simulink model "modelo_planta_CODESYS"  (R2025b)
settings: Solver=FixedStepAuto  StartTime=0.0  StopTime=inf  FixedStep=Ts2  MaxStep=1e-3  RelTol=1e-3
undefined symbols (not defined in the file): ah_max, at_max, bcx, bcy, bh_eq, bhb, bhEb, bhwu, bt, bt_eq, btb, btw, g, Hc, ih, it, Jh_eq, Jt_eq, Kcy, khwu, Ki_h, Ki_t, Kp_h, Kp_t, Kpos_h, Kpos_t, Ktw, lambda, Lh, Lh0, lh_0, Lt, magnitude, Mc_max, Ms, Mt, rhd, rtd, tau_hm, tau_tm, Thb_Max, ThEb_Max, Thm_0, Thm_Max, titahm_0, titatm_0, Ts0, Ts1, Ts2, Ttb_Max, Ttm_0, Ttm_Max, vh_0, vlx_0, vly_0, vt_0, vt_max, Wc, whm_0, whm_rated ... (+11)
libraries: simulink x10, opcualib x7, sl3dlib x1, simulink_extras x1, dspnetwork x1
(part 2 of 2)

== system modelo_planta_CODESYS/Subsistema Izaje/Dinámica carga izaje/Lógica Masa y Altura ==
  McX : Inport
  TLK : Inport  Port=2
  Constant : Constant  Value=Ms
  Constant1 : Constant  Value=0
  Constant2 : Constant  Value=Hc
  Rate Limiter : RateLimiter  Commented=through  RisingSlewLimit=Mc_max/0.1  FallingSlewLimit=-Mc_max/0.1  SampleTimeMode=inherited  InitialCondition=Ms
  Sum1 : Sum  Inputs=|++
  Switch : Switch  Criteria=u2 > Threshold  SaturateOnIntegerOverflow=off  InputSameDT=off
  Switch1 : Switch  Criteria=u2 > Threshold  SaturateOnIntegerOverflow=off  InputSameDT=off
  ml : Outport
  hc : Outport  Port=2
  wires:
  Sum1/1 -> Switch/1
  Constant2/1 -> Switch1/1
  TLK/1 -> Switch1/2, Switch/2
  Constant/1 -> Switch/3, Sum1/2
  Constant1/1 -> Switch1/3
  McX/1 -> Sum1/1
  Switch/1 -> Rate Limiter/1
  Rate Limiter/1 -> ml/1
  Switch1/1 -> hc/1

== system modelo_planta_CODESYS/Subsistema Izaje/Dinámica carga izaje/Lógica contacto ==
  delta_y : Inport
  vlx : Inport  Port=2
  vly : Inport  Port=3
  Constant3 : Constant  Value=0
  Constant4 : Constant  Value=0
  Gain3 : Gain  Gain=Kcy
  Gain4 : Gain  Gain=bcy
  Gain5 : Gain  Gain=-bcx
  Saturation : Saturate  UpperLimit=60e5  LowerLimit=0
  Sum5 : Sum  Inputs=-+|
  Switch2 : Switch  SaturateOnIntegerOverflow=off  InputSameDT=off
  Switch3 : Switch  SaturateOnIntegerOverflow=off  InputSameDT=off
  Fcy : Outport
  Fcx : Outport  Port=2
  wires:
  Sum5/1 -> Switch2/1
  vlx/1 -> Gain5/1
  Gain4/1 -> Sum5/1
  vly/1 -> Gain4/1
  Constant4/1 -> Switch3/3
  Gain5/1 -> Switch3/1
  Gain3/1 -> Sum5/2
  delta_y/1 -> Switch3/2, Gain3/1, Switch2/2
  Constant3/1 -> Switch2/3
  Switch2/1 -> Saturation/1  "Fcy"
  Switch3/1 -> Fcx/1  "Fcx"
  Saturation/1 -> Fcy/1

== matlab function modelo_planta_CODESYS/Controlador Carro v2/MATLAB Function ==
  data: tita_l input; v_sway output; yh_enc input; m_est input; Yt0 parameter; g parameter; lambda parameter; Ms parameter; Mc_max parameter; antisway input
function v_sway = Control_Balanceo(tita_l, yh_enc, m_est, Yt0, g, lambda, Ms, Mc_max, antisway)
    
    % 1. Compensación de inercia (ganancia_masa)
    L_vacio = 1.0;
    L_lleno = 0.6;
    
    factor = (m_est - Ms) / Mc_max;
    factor = max(0, min(1, factor)); % Saturación entre 0 y 1
    
    g_masa = L_vacio + (L_lleno - L_vacio) * factor;

    % 2. Cinemática del péndulo
    % Longitud del cable (l)
    l_pendulo = Yt0 - yh_enc;
    
    % Ganancia cinemática
    K_cinematico = 2 * lambda * g_masa * sqrt(abs(g * l_pendulo));

    % 3. Multiplicación por el ángulo y activación del bloque
    v_sway = tita_l * K_cinematico * antisway;
end

== matlab function modelo_planta_CODESYS/Controlador Carro v2/MATLAB Function1 ==
  data: x_ref_s output; xt_ref input; vt_max parameter; at_max parameter; v_ref_s output; Ts2 parameter; xt_0 parameter; vt_0 parameter
function [x_ref_s, v_ref_s] = Curva_S_t(xt_ref, vt_max, at_max, Ts2, xt_0, vt_0)
    % Memorias (Equivalente a los bloques Z^-1)
    persistent x_ref_s_prev v_ref_s_prev
    
    % Inicialización en el primer ciclo
    if isempty(x_ref_s_prev)
        x_ref_s_prev = xt_0;
        v_ref_s_prev = vt_0;
    end
    
    % 1. Sumador de entrada (Error de posición)
    error_pos = xt_ref - x_ref_s_prev;
    
    % 2. Frenado Óptimo
    d_tol = 0.1;
    if abs(error_pos) > d_tol
        vh_brakes = sqrt(2 * at_max * abs(error_pos));
        vt_cmd = vh_brakes * sign(error_pos);
    else
        vh_limit_tol = sqrt(2 * at_max * d_tol);
        gain_linear = vh_limit_tol / d_tol;      
        vt_cmd = gain_linear * error_pos;
    end
    
    % 3. Saturación (Limitar la velocidad máxima)
    vt_cmd_sat = max(-vt_max, min(vt_max, vt_cmd));
    
    % 4. Rate Limiter
    delta_v = vt_cmd_sat - v_ref_s_prev;
    limite_delta = at_max * Ts2; % Cuánto puede cambiar la velocidad en 1 ciclo
    
    delta_v_limitado = max(-limite_delta, min(limite_delta, delta_v));
    v_ref_s = v_ref_s_prev + delta_v_limitado;
    
    % 5. Integrador Discreto (Tustin)
    x_ref_s = x_ref_s_prev + (Ts2 / 2) * (v_ref_s + v_ref_s_prev);
    
    % 6. Actualizar memorias para el siguiente ciclo
    v_ref_s_prev = v_ref_s;
    x_ref_s_prev = x_ref_s;
end

== matlab function modelo_planta_CODESYS/Controlador Carro v2/MATLAB Function2 ==
  data: vx_cmd input; vt_ref output; modo_manual input; x_ref_s input; v_ref_s input; xtd_enc input; v_sway input; vt_0 parameter; Ts2 parameter; at_max parameter; vt_max parameter; Kpos_t parameter
function vt_ref = Lazo_Externo_t(vx_cmd, modo_manual, x_ref_s, v_ref_s, xtd_enc, v_sway, vt_0, Ts2, at_max, vt_max, Kpos_t)
    % Memoria
    persistent vt_ref_prev
    
    if isempty(vt_ref_prev)
        vt_ref_prev = vt_0;
    end

    % 1. Control de posición automático
    e_x = x_ref_s - xtd_enc;
    vel_auto = (e_x * Kpos_t) + (v_ref_s * 0.5);

    % 2. Selector de Modo
    % Si modo_manual es true (1), pasa la señal manual, si no, la automática
    if modo_manual > 0 
        vel_base = vx_cmd;
    else
        vel_base = vel_auto;
    end

    % 3. Suma del Anti-Sway
    vt_cmd = vel_base + v_sway;

    % 4. Límite de Velocidad
    vt_cmd_sat = max(-vt_max, min(vt_max, vt_cmd));

    % 5. Límite de Aceleración
    delta_v = vt_cmd_sat - vt_ref_prev;
    limite_delta = at_max * Ts2;
    
    delta_v_limitado = max(-limite_delta, min(limite_delta, delta_v));
    vt_ref = vt_ref_prev + delta_v_limitado;

    % 6. Actualizar memoria
    vt_ref_prev = vt_ref;
end

== matlab function modelo_planta_CODESYS/Controlador Carro v2/MATLAB Function3 ==
  data: xtd_enc input; vt_obs output; Ttm_ref input; wtm_0 parameter; titatm_0 parameter; Lt parameter; bt_eq parameter; Jt_eq parameter; rtd parameter; it parameter; Ts2 parameter
function vt_obs = Observador_Estado_t(xtd_enc, Ttm_ref, wtm_0, titatm_0, Lt, bt_eq, Jt_eq, rtd, it, Ts2)...
    
    % Memorias
    persistent theta_t_obs_prev wt_obs_prev int_e_prev
    
    % Condiciones iniciales
    if isempty(theta_t_obs_prev)
        theta_t_obs_prev = titatm_0;
        wt_obs_prev      = wtm_0;    
        int_e_prev       = 0.0; 
    end
    
    % 1. Convertir posición lineal del carro a angular del motor
    theta_t_enc = xtd_enc * (it / rtd);
    
    % 2. Error de estimación (Posición real vs observada)
    e_theta_t = theta_t_enc - theta_t_obs_prev;
    
    % 3. Lazo de torque (Física de la planta)
    Torque_net = Ttm_ref - (bt_eq * wt_obs_prev) + (Lt(3) * int_e_prev);
    alpha_phys = Torque_net / Jt_eq; % Aceleración angular
    
    % 4. Derivadas
    dot_wt_obs      = alpha_phys + (Lt(2) * e_theta_t);
    dot_theta_t_obs = wt_obs_prev + (Lt(1) * e_theta_t);

    % 5. Salida del observador
    vt_obs = wt_obs_prev * (rtd / it);
    
    % 6. Integración Discreta
    theta_t_obs = theta_t_obs_prev + (Ts2 * dot_theta_t_obs);
    wt_obs      = wt_obs_prev      + (Ts2 * dot_wt_obs);
    int_e       = int_e_prev       + (Ts2 * e_theta_t);

    % 7. Actualizar memorias para el siguiente ciclo de reloj
    theta_t_obs_prev = theta_t_obs;
    wt_obs_prev      = wt_obs;
    int_e_prev       = int_e;
end

== matlab function modelo_planta_CODESYS/Controlador Carro v2/MATLAB Function4 ==
  data: vt_ref input; Ttm_ref output; vt_obs input; BRK_t input; Ts2 parameter; Ki_t parameter; Kp_t parameter
function Ttm_ref = Lazo_Interno_t(vt_ref, vt_obs, BRK_t, Ts2, Ki_t, Kp_t)
    % Memorias para el integrador
    persistent int_prev e_v_prev
    
    % Inicialización
    if isempty(int_prev)
        int_prev = 0.0;
        e_v_prev = 0.0;
    end
    
    % 1. Cálculo del error de velocidad
    e_v = vt_ref - vt_obs;
    
    % 2. Integrador Discreto (Tustin) con Reset por Freno
    % Si el freno está activo (BRK_t = 0), forzamos la memoria a 0 
    % para evitar la acumulación de error (Anti-Windup).
    if BRK_t > 0
        int_val = int_prev + (Ts2 / 2) * (e_v + e_v_prev);
    else
        int_val = 0.0;
    end
    
    % 3. Controlador PI
    P_out = e_v * Kp_t;
    I_out = int_val * Ki_t;
    
    % Suma final de referencia de torque
    Ttm_ref = P_out + I_out;
    
    % 4. Actualizar memorias
    int_prev = int_val;
    e_v_prev = e_v;
end

== matlab function modelo_planta_CODESYS/Controlador Izaje v2/MATLAB Function1 ==
  data: y_ref_s output; yh_ref input; ah_max parameter; v_ref_s output; Ts2 parameter; yh_0 parameter; vh_0 parameter; vh_lim input
function [y_ref_s, v_ref_s] = Curva_S_h(yh_ref, ah_max, Ts2, yh_0, vh_0, vh_lim)
    % Memorias (Equivalente a los bloques Z^-1)
    persistent x_ref_s_prev v_ref_s_prev
    
    % Inicialización en el primer ciclo
    if isempty(x_ref_s_prev)
        x_ref_s_prev = yh_0;
        v_ref_s_prev = vh_0;
    end
    
    % 1. Sumador de entrada (Error de posición)
    error_pos = yh_ref - x_ref_s_prev;
    
    % 2. Frenado Óptimo
    d_tol = 0.1;
    if abs(error_pos) > d_tol
        vh_brakes = sqrt(2 * ah_max * abs(error_pos));
        vt_cmd = vh_brakes * sign(error_pos);
    else
        vh_limit_tol = sqrt(2 * ah_max * d_tol);
        gain_linear = vh_limit_tol / d_tol;      
        vt_cmd = gain_linear * error_pos;
    end
    
    % 3. Saturación (Limitar la velocidad máxima)
    vt_cmd_sat = max(-vh_lim, min(vh_lim, vt_cmd));
    
    % 4. Rate Limiter
    delta_v = vt_cmd_sat - v_ref_s_prev;
    limite_delta = ah_max * Ts2; % Cuánto puede cambiar la velocidad en 1 ciclo
    
    delta_v_limitado = max(-limite_delta, min(limite_delta, delta_v));
    v_ref_s = v_ref_s_prev + delta_v_limitado;
    
    % 5. Integrador Discreto (Tustin)
    y_ref_s = x_ref_s_prev + (Ts2 / 2) * (v_ref_s + v_ref_s_prev);
    
    % 6. Actualizar memorias para el siguiente ciclo
    v_ref_s_prev = v_ref_s;
    x_ref_s_prev = y_ref_s;
end

== matlab function modelo_planta_CODESYS/Controlador Izaje v2/MATLAB Function2 ==
  data: vy_cmd input; modo_manual input; y_ref_s input; v_ref_s input; vh_lim input; yh_enc input; vh_ref output; Ts2 parameter; ah_max parameter; Kpos_h parameter; vh_0 parameter
function vh_ref = Lazo_Externo_h(vy_cmd, modo_manual, y_ref_s, v_ref_s, vh_lim, yh_enc, Ts2, ah_max, Kpos_h, vh_0)
    % Memoria
    persistent vh_ref_prev
    
    if isempty(vh_ref_prev)
        vh_ref_prev = vh_0;
    end

    % 1. Control de posición automático
    e_y = y_ref_s - yh_enc;
    vel_auto = (e_y * Kpos_h) + (v_ref_s * 0.5);

    % 2. Selector de Modo
    % Si modo_manual es true (1), pasa la señal manual, si no, la automática
    if modo_manual > 0 
        vh_cmd = vy_cmd;
    else
        vh_cmd = vel_auto;
    end

    % 3. Límite de Velocidad
    vh_cmd_sat = max(-vh_lim, min(vh_lim, vh_cmd));

    % 5. Límite de Aceleración
    delta_v = vh_cmd_sat - vh_ref_prev;
    limite_delta = ah_max * Ts2;
    
    delta_v_limitado = max(-limite_delta, min(limite_delta, delta_v));
    vh_ref = vh_ref_prev + delta_v_limitado;

    % 6. Actualizar memoria
    vh_ref_prev = vh_ref;
end

== matlab function modelo_planta_CODESYS/MATLAB Function ==
  data: TLK input; M_carga output; Mc_min parameter
function M_carga = Masa_Aleatoria(TLK, Mc_min)
    persistent masa_actual;
    persistent ultimo_estado_trigger;
    
    % Inicialización
    if isempty(masa_actual)
        masa_actual = Mc_min; % Empezamos con el valor mínimo por defecto
        ultimo_estado_trigger = 0;
    end
    
    % DETECCIÓN DE FLANCO DE SUBIDA (Rising Edge)
    if (TLK == 1 && ultimo_estado_trigger == 0)
        % Generar número aleatorio entre Min y Max
        masa_actual = Mc_min + (55000 - Mc_min) * rand();
        masa_actual = floor(masa_actual); 
    end
    
    % Actualizar memoria del trigger
    ultimo_estado_trigger = TLK;
    % Salida: La masa se mantiene constante hasta el próximo trigger
    M_carga = masa_actual;
end

== matlab function modelo_planta_CODESYS/Controlador Izaje v2/MATLAB Function3 ==
  data: yh_enc input; vh_obs output; Thm_ref input; whm_0 parameter; titahm_0 parameter; Lh parameter; bh_eq parameter; Jh_eq parameter; rhd parameter; ih parameter; Ts2 parameter; Ms parameter; g parameter
function vh_obs = Observador_Estado_h(yh_enc, Thm_ref, whm_0, titahm_0,...
    Lh, bh_eq, Jh_eq, rhd, ih, Ts2, Ms, g)
    
    % Memorias
    persistent theta_h_obs_prev wh_obs_prev int_e_prev
    
    % Condiciones iniciales
    if isempty(theta_h_obs_prev)
        theta_h_obs_prev = titahm_0;
        wh_obs_prev      = whm_0;    
        int_e_prev       = 0.0; 
    end
    
    % 1. Convertir posición lineal del carro a angular del motor
    theta_h_enc = yh_enc * (2*ih / rhd);
    
    % 2. Error de estimación (Posición real vs observada)
    e_theta_h = theta_h_enc - theta_h_obs_prev;
    
    % 3. Lazo de torque (Física de la planta)
    Torque_net = Thm_ref - (Ms*g*rhd/(2*ih)) - (bh_eq * wh_obs_prev) +...
        (Lh(3) * int_e_prev);
    alpha_phys = Torque_net / Jh_eq; % Aceleración angular
    
    % 4. Derivadas
    dot_wh_obs      = alpha_phys + (Lh(2) * e_theta_h);
    dot_theta_h_obs = wh_obs_prev + (Lh(1) * e_theta_h);

    % 5. Salida del observador
    vh_obs = wh_obs_prev * (rhd / (2*ih));
    
    % 6. Integración Discreta
    theta_h_obs = theta_h_obs_prev + (Ts2 * dot_theta_h_obs);
    wh_obs      = wh_obs_prev      + (Ts2 * dot_wh_obs);
    int_e       = int_e_prev       + (Ts2 * e_theta_h);

    % 7. Actualizar memorias para el siguiente ciclo de reloj
    theta_h_obs_prev = theta_h_obs;
    wh_obs_prev      = wh_obs;
    int_e_prev       = int_e;
end

== matlab function modelo_planta_CODESYS/Controlador Izaje v2/MATLAB Function4 ==
  data: m_est input; vh_ref input; Thm_ref output; vh_obs input; BRK_h input; BRK_hE input; Ts2 parameter; Ki_h parameter; Kp_h parameter; g parameter; rhd parameter; ih parameter
function Thm_ref = Lazo_Interno_h(m_est, vh_ref, vh_obs, BRK_h, BRK_hE, Ts2, Ki_h, Kp_h, g, rhd, ih)
    % Memorias para el integrador
    persistent int_prev e_w_prev
    
    % Inicialización
    if isempty(int_prev)
        int_prev = 0.0;
        e_w_prev = 0.0;
    end
    
    % 1. Cálculo del error de velocidad angular
    e_w = (vh_ref - vh_obs) * (2*ih/rhd);
    
    % 2. Integrador Discreto (Tustin) con Reset por Freno
    % Si el freno está activo (BRK_h = 0 || BRK_hE = 0), forzamos la 
    % memoria a 0 para evitar la acumulación de error (Anti-Windup).
    if BRK_h > 0 && BRK_hE > 0
        int_val = int_prev + (Ts2 / 2) * (e_w + e_w_prev);
    else
        int_val = 0.0;
    end
    
    % 3. Controlador PI + Feedfoward de gravedad
    P_out = e_w * Kp_h;
    I_out = int_val * Ki_h;
    Tg_ff = m_est * (g*rhd/(2*ih));
    
    % Suma final de referencia de torque
    Thm_ref = P_out + I_out + Tg_ff;
    
    % 4. Actualizar memorias
    int_prev = int_val;
    e_w_prev = e_w;
end

== matlab function modelo_planta_CODESYS/MATLAB Function1 ==
  data: yc0 output; xl input; xt_min parameter; Wc parameter; h_vec input
function yc0 = Y_spreader(xl, xt_min, Wc, h_vec)
% Cálculo índice de spreader
i_spreader = floor((xl - xt_min)/Wc) + 1;
i_spreader = min(max(i_spreader, 1), 33);

% Obtención de yc0 usando la posición del spreader
yc0 = h_vec(i_spreader);
